simulink subsystem "ros_command"  (R2022a)
settings: Solver=VariableStepAuto  StartTime=0.0  StopTime=10.0  RelTol=1e-3
undefined symbols (not defined in the file): MPC, simulink
libraries: robotlib x42
settings Model: Creator=lamarre  LastModifiedBy=lamarre
settings DebuggingCC: UnconnectedInputMsg=warning  UnconnectedOutputMsg=warning  UnconnectedLineMsg=warning
settings RTWCC: DLArmComputeVersion=19.05

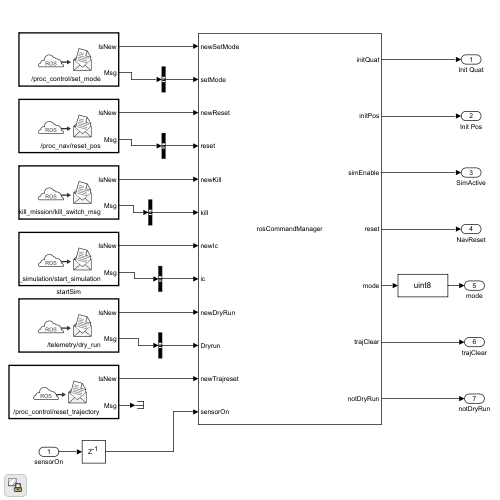
[thumbnail: Simulink's stored preview of the top-level diagram]
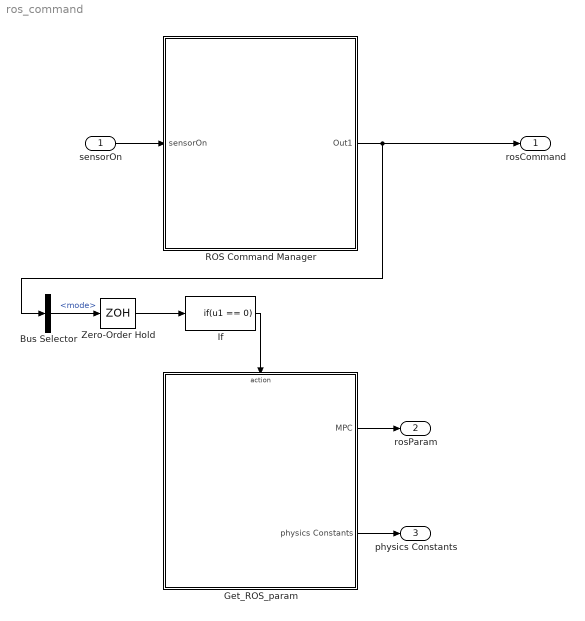
== system ros_command ==
  sensorOn : Inport
  Bus Selector : BusSelector  OutputSignals=mode
  "Get_ROS_param " : Subsystem
  If : If  IfExpression=u1 == 0  ShowElse=off
  ROS Command Manager : Subsystem  TreatAsAtomicUnit=on  SystemSampleTime=MPC.Ts
  Zero-Order Hold : ZeroOrderHold  SampleTime=simulink.ros.paramSampletime
  rosCommand : Outport
  rosParam : Outport  Port=2
  physics Constants : Outport  Port=3
  wires:
  sensorOn/1 -> ROS Command Manager/1(sensorOn)
  ROS Command Manager/1(Out1) -> rosCommand/1, Bus Selector/1
  If/1 -> "Get_ROS_param "/Action
  Bus Selector/1 -> Zero-Order Hold/1  "<mode>"
  "Get_ROS_param "/1(MPC) -> rosParam/1
  "Get_ROS_param "/2(physics Constants) -> physics Constants/1
  Zero-Order Hold/1 -> If/1

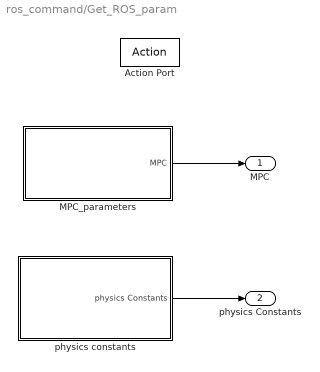
== system ros_command/Get_ROS_param  ==
  Action Port : ActionPort  InitializeStates=reset
  MPC_parameters : Subsystem
  physics constants : Subsystem
  MPC : Outport
  physics Constants : Outport  Port=2
  wires:
  physics constants/1(physics Constants) -> physics Constants/1
  MPC_parameters/1(MPC) -> MPC/1

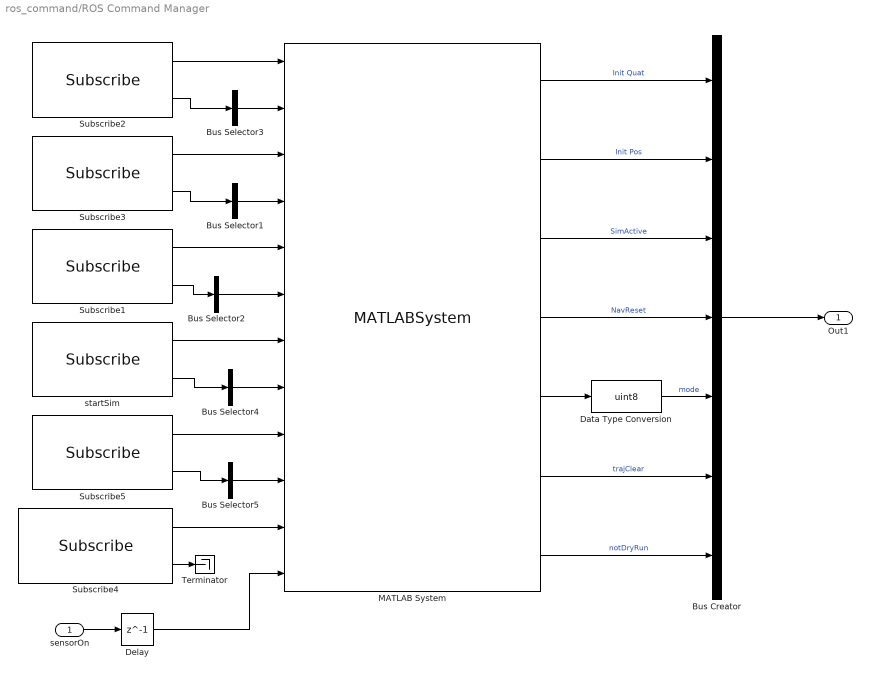
== system ros_command/ROS Command Manager ==
  sensorOn : Inport
  Bus Creator : BusCreator  Inputs=7
  Bus Selector{1..3,5} (4 alike) : BusSelector  OutputSignals=Data  OutputAsBus=on
  Bus Selector4 : BusSelector  OutputSignals=Position.X,Position.Y,Position.Z,Orientation.W,Orientation.X,Orientation.Y,Orientation.Z  OutputAsBus=on
  Data Type Conversion : DataTypeConversion  OutDataTypeStr=uint8  SaturateOnIntegerOverflow=off  RndMeth=Floor
  Delay : Delay  DelayLength=1  InitialCondition=0
  MATLAB System : MATLABSystem  System=rosCommandManager  initial_mode=mode.init  SimulateUsing=Code generation
      mask Type: rosCommandManager
      mask Display:
      | disp('rosCommandManager');
      | port_label('input',1,'newSetMode');
      | port_label('input',2,'setMode');
      | port_label('input',3,'newReset');
      | port_label('input',4,'reset');
      | port_label('input',5,'newKill');
      | port_label('input',6,'kill');
      | port_label('input',7,'newIc');
      | port_label('input',8,'ic');
      | port_label('input',9,'newDryRun');
      | port_label('input',10,'Dryrun');
      | port_label('input',11,'newTrajreset');
      | port_label('input',12,'sensorOn');
      | port_label('output',1,'initQuat');
      | port_label('output',2,'initPos');
      | port_label('output',3,'simEnable');
      | port_label('output',4,'reset');
      | port_label('output',5,'mode');
      | port_label('output',6,'trajClear');
      | port_label('output',7,'notDryRun');
  Subscribe1 : robotlib/Subscribe  topicSource=Specify your own  topic=/provider_kill_mission/kill_switch_msg  messageType=std_msgs/Bool  SampleTime=MPC.Ts  legacyBusStruct=off  messageQueueLength=1
  Subscribe2 : robotlib/Subscribe  topicSource=Specify your own  topic=/proc_control/set_mode  messageType=std_msgs/UInt8  SampleTime=MPC.Ts  legacyBusStruct=off  messageQueueLength=1
  Subscribe3 : robotlib/Subscribe  topicSource=Specify your own  topic=/proc_nav/reset_pos  messageType=std_msgs/Bool  SampleTime=MPC.Ts  legacyBusStruct=off  messageQueueLength=1
  Subscribe4 : robotlib/Subscribe  topicSource=Specify your own  topic=/proc_control/reset_trajectory  messageType=std_msgs/Bool  SampleTime=MPC.Ts  legacyBusStruct=off  messageQueueLength=1
  Subscribe5 : robotlib/Subscribe  topicSource=Specify your own  topic=/telemetry/dry_run  messageType=std_msgs/Bool  SampleTime=MPC.Ts  legacyBusStruct=off  messageQueueLength=1
  Terminator : Terminator
  startSim : robotlib/Subscribe  topicSource=Specify your own  topic=/proc_simulation/start_simulation  messageType=geometry_msgs/Pose  SampleTime=MPC.Ts  legacyBusStruct=off  messageQueueLength=1
  Out1 : Outport
  wires:
  Subscribe3/1 -> MATLAB System/3
  Bus Selector5/1 -> MATLAB System/10
  startSim/2 -> Bus Selector4/1
  Subscribe2/1 -> MATLAB System/1
  MATLAB System/4 -> Bus Creator/4  "NavReset"
  Subscribe4/1 -> MATLAB System/11
  Bus Selector2/1 -> MATLAB System/6
  Bus Creator/1 -> Out1/1
  Bus Selector4/1 -> MATLAB System/8
  Subscribe3/2 -> Bus Selector1/1
  MATLAB System/7 -> Bus Creator/7  "notDryRun"
  Data Type Conversion/1 -> Bus Creator/5  "mode"
  sensorOn/1 -> Delay/1
  Subscribe4/2 -> Terminator/1
  Bus Selector3/1 -> MATLAB System/2
  startSim/1 -> MATLAB System/7
  MATLAB System/3 -> Bus Creator/3  "SimActive"
  Subscribe5/2 -> Bus Selector5/1
  Subscribe1/1 -> MATLAB System/5
  Subscribe2/2 -> Bus Selector3/1
  Subscribe1/2 -> Bus Selector2/1
  Bus Selector1/1 -> MATLAB System/4
  Delay/1 -> MATLAB System/12
  Subscribe5/1 -> MATLAB System/9
  MATLAB System/6 -> Bus Creator/6  "trajClear"
  MATLAB System/2 -> Bus Creator/2  "Init Pos"
  MATLAB System/5 -> Data Type Conversion/1
  MATLAB System/1 -> Bus Creator/1  "Init Quat"

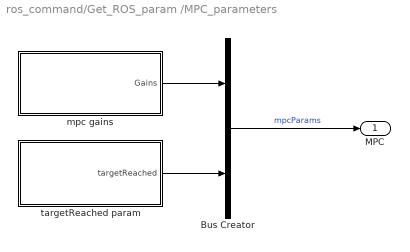
== system ros_command/Get_ROS_param /MPC_parameters ==
  Bus Creator : BusCreator  Inputs=2  OutDataTypeStr=Bus: mpcParams  NonVirtualBus=on
  mpc gains : Subsystem
  targetReached param : Subsystem
  MPC : Outport
  wires:
  Bus Creator/1 -> MPC/1  "mpcParams"
  mpc gains/1(Gains) -> Bus Creator/1
  targetReached param/1(targetReached) -> Bus Creator/2

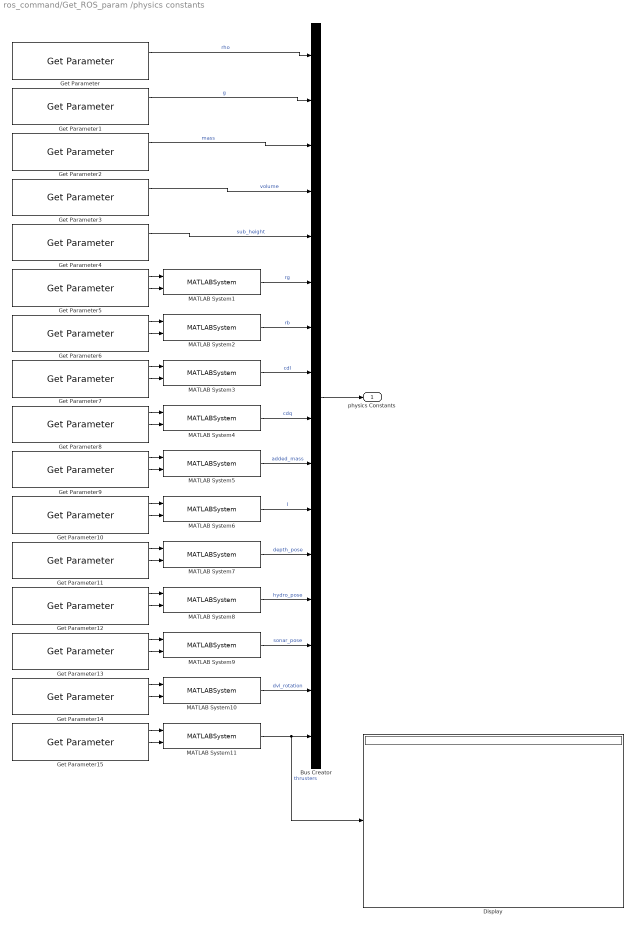
== system ros_command/Get_ROS_param /physics constants ==
  Bus Creator : BusCreator  Inputs=16  OutDataTypeStr=Bus: physicsConstants  NonVirtualBus=on
  Display : Display
  Get Parameter : robotlib/Get Parameter  ParameterSource=Specify your own  ParameterName=/proc_control/physics/rho  ParameterType=double  ParameterMaxArrayLength=16  ParameterInitialValue=physics.rho  SampleTime=-1  ShowErrorCodeOutput=on  ModelName=proc_control  BlockId=ParamGet_proc_control_185_535
      settings: SourceProductBaseCode=RR
  Get Parameter1 : robotlib/Get Parameter  ParameterSource=Specify your own  ParameterName=/proc_control/physics/g  ParameterType=double  ParameterMaxArrayLength=16  ParameterInitialValue=physics.g  SampleTime=-1  ShowErrorCodeOutput=on  ModelName=proc_control  BlockId=ParamGet_proc_control_185_540
      settings: SourceProductBaseCode=RR
  Get Parameter10 : robotlib/Get Parameter  ParameterSource=Specify your own  ParameterName=/proc_control/physics/I  ParameterType=uint8[] (string)  ParameterMaxArrayLength=128  ParameterInitialValue=int8('0,0,0,0,0,0,0,0,0')  SampleTime=-1  ShowErrorCodeOutput=on  ModelName=proc_control  BlockId=ParamGet_proc_control_185_554
      settings: SourceProductBaseCode=RR
  Get Parameter11 : robotlib/Get Parameter  ParameterSource=Specify your own  ParameterName=/proc_control/physics/depth_pose  ParameterType=uint8[] (string)  ParameterMaxArrayLength=64  ParameterInitialValue=int8('0,0,0')  SampleTime=-1  ShowErrorCodeOutput=on  ModelName=proc_control  BlockId=ParamGet_proc_control_185_556
      settings: SourceProductBaseCode=RR
  Get Parameter12 : robotlib/Get Parameter  ParameterSource=Specify your own  ParameterName=/proc_control/physics/hydro_pose  ParameterType=uint8[] (string)  ParameterMaxArrayLength=64  ParameterInitialValue=int8('0,0,0')  SampleTime=-1  ShowErrorCodeOutput=on  ModelName=proc_control  BlockId=ParamGet_proc_control_185_558
      settings: SourceProductBaseCode=RR
  Get Parameter13 : robotlib/Get Parameter  ParameterSource=Specify your own  ParameterName=/proc_control/physics/sonar_pose  ParameterType=uint8[] (string)  ParameterMaxArrayLength=64  ParameterInitialValue=int8('0,0,0')  SampleTime=-1  ShowErrorCodeOutput=on  ModelName=proc_control  BlockId=ParamGet_proc_control_185_560
      settings: SourceProductBaseCode=RR
  Get Parameter14 : robotlib/Get Parameter  ParameterSource=Specify your own  ParameterName=/proc_control/physics/dvl_rotation  ParameterType=uint8[] (string)  ParameterMaxArrayLength=64  ParameterInitialValue=int8('0,0,0')  SampleTime=-1  ShowErrorCodeOutput=on  ModelName=proc_control  BlockId=ParamGet_proc_control_185_562
      settings: SourceProductBaseCode=RR
  Get Parameter15 : robotlib/Get Parameter  ParameterSource=Specify your own  ParameterName=/proc_control/physics/thrusters  ParameterType=uint8[] (string)  ParameterMaxArrayLength=400  ParameterInitialValue=int8('0,0,0')  SampleTime=-1  ShowErrorCodeOutput=on  ModelName=proc_control  BlockId=ParamGet_proc_control_185_568
      settings: SourceProductBaseCode=RR
  Get Parameter2 : robotlib/Get Parameter  ParameterSource=Specify your own  ParameterName=/proc_control/physics/mass  ParameterType=double  ParameterMaxArrayLength=16  ParameterInitialValue=physics.mass  SampleTime=-1  ShowErrorCodeOutput=on  ModelName=proc_control  BlockId=ParamGet_proc_control_185_541
      settings: SourceProductBaseCode=RR
  Get Parameter3 : robotlib/Get Parameter  ParameterSource=Specify your own  ParameterName=/proc_control/physics/volume  ParameterType=double  ParameterMaxArrayLength=16  ParameterInitialValue=physics.volume  SampleTime=-1  ShowErrorCodeOutput=on  ModelName=proc_control  BlockId=ParamGet_proc_control_185_542
      settings: SourceProductBaseCode=RR
  Get Parameter4 : robotlib/Get Parameter  ParameterSource=Specify your own  ParameterName=/proc_control/physics/sub_height  ParameterType=double  ParameterMaxArrayLength=16  ParameterInitialValue=physics.height  SampleTime=-1  ShowErrorCodeOutput=on  ModelName=proc_control  BlockId=ParamGet_proc_control_185_543
      settings: SourceProductBaseCode=RR
  Get Parameter5 : robotlib/Get Parameter  ParameterSource=Specify your own  ParameterName=/proc_control/physics/rg  ParameterType=uint8[] (string)  ParameterMaxArrayLength=64  ParameterInitialValue=int8('0,0,0')  SampleTime=-1  ShowErrorCodeOutput=on  ModelName=proc_control  BlockId=ParamGet_proc_control_185_544
      settings: SourceProductBaseCode=RR
  Get Parameter6 : robotlib/Get Parameter  ParameterSource=Specify your own  ParameterName=/proc_control/physics/rb  ParameterType=uint8[] (string)  ParameterMaxArrayLength=64  ParameterInitialValue=int8('0,0,0')  SampleTime=-1  ShowErrorCodeOutput=on  ModelName=proc_control  BlockId=ParamGet_proc_control_185_546
      settings: SourceProductBaseCode=RR
  Get Parameter7 : robotlib/Get Parameter  ParameterSource=Specify your own  ParameterName=/proc_control/physics/cdl  ParameterType=uint8[] (string)  ParameterMaxArrayLength=64  ParameterInitialValue=int8('0,0,0,0,0,0')  SampleTime=-1  ShowErrorCodeOutput=on  ModelName=proc_control  BlockId=ParamGet_proc_control_185_548
      settings: SourceProductBaseCode=RR
  Get Parameter8 : robotlib/Get Parameter  ParameterSource=Specify your own  ParameterName=/proc_control/physics/cdq  ParameterType=uint8[] (string)  ParameterMaxArrayLength=64  ParameterInitialValue=int8('0,0,0,0,0,0')  SampleTime=-1  ShowErrorCodeOutput=on  ModelName=proc_control  BlockId=ParamGet_proc_control_185_549
      settings: SourceProductBaseCode=RR
  Get Parameter9 : robotlib/Get Parameter  ParameterSource=Specify your own  ParameterName=/proc_control/physics/added_mass  ParameterType=uint8[] (string)  ParameterMaxArrayLength=64  ParameterInitialValue=int8('0,0,0,0,0,0')  SampleTime=-1  ShowErrorCodeOutput=on  ModelName=proc_control  BlockId=ParamGet_proc_control_185_552
      settings: SourceProductBaseCode=RR
  MATLAB System1 : MATLABSystem  System=String2DoubleArray  arraySize=[1, 3]  constantName='Center of mass'  SimulateUsing=Code generation
      mask Type: String2DoubleArray
      mask Display:
      | disp('String2DoubleArray');
      | port_label('input',1,'string');
      | port_label('input',2,'length');
      | port_label('output',1,'array');
  MATLAB System10 : MATLABSystem  System=String2DoubleArray  arraySize=[1, 3]  constantName='DVL Rotation'  SimulateUsing=Code generation
      mask Type: String2DoubleArray
      mask Display:
      | disp('String2DoubleArray');
      | port_label('input',1,'string');
      | port_label('input',2,'length');
      | port_label('output',1,'array');
  MATLAB System11 : MATLABSystem  System=String2DoubleArray  arraySize=[MPC.nu 6]  constantName='Thrusters Config'  SimulateUsing=Code generation
      mask Type: String2DoubleArray
      mask Display:
      | disp('String2DoubleArray');
      | port_label('input',1,'string');
      | port_label('input',2,'length');
      | port_label('output',1,'array');
  MATLAB System2 : MATLABSystem  System=String2DoubleArray  arraySize=[1, 3]  constantName='Center of buoyancy'  SimulateUsing=Code generation
      mask Type: String2DoubleArray
      mask Display:
      | disp('String2DoubleArray');
      | port_label('input',1,'string');
      | port_label('input',2,'length');
      | port_label('output',1,'array');
  MATLAB System3 : MATLABSystem  System=String2DoubleArray  arraySize=[1,6]  constantName='Linear drag constants'  SimulateUsing=Code generation
      mask Type: String2DoubleArray
      mask Display:
      | disp('String2DoubleArray');
      | port_label('input',1,'string');
      | port_label('input',2,'length');
      | port_label('output',1,'array');
  MATLAB System4 : MATLABSystem  System=String2DoubleArray  arraySize=[1, 6]  constantName='Quadratic drag constants'  SimulateUsing=Code generation
      mask Type: String2DoubleArray
      mask Display:
      | disp('String2DoubleArray');
      | port_label('input',1,'string');
      | port_label('input',2,'length');
      | port_label('output',1,'array');
  MATLAB System5 : MATLABSystem  System=String2DoubleArray  arraySize=[1, 6]  constantName='Added Mass'  SimulateUsing=Code generation
      mask Type: String2DoubleArray
      mask Display:
      | disp('String2DoubleArray');
      | port_label('input',1,'string');
      | port_label('input',2,'length');
      | port_label('output',1,'array');
  MATLAB System6 : MATLABSystem  System=String2DoubleArray  arraySize=[1,9]  constantName='Inertia Tensor'  SimulateUsing=Code generation
      mask Type: String2DoubleArray
      mask Display:
      | disp('String2DoubleArray');
      | port_label('input',1,'string');
      | port_label('input',2,'length');
      | port_label('output',1,'array');
  MATLAB System7 : MATLABSystem  System=String2DoubleArray  arraySize=[1, 3]  constantName='Depth Pose'  SimulateUsing=Code generation
      mask Type: String2DoubleArray
      mask Display:
      | disp('String2DoubleArray');
      | port_label('input',1,'string');
      | port_label('input',2,'length');
      | port_label('output',1,'array');
  MATLAB System8 : MATLABSystem  System=String2DoubleArray  arraySize=[1, 3]  constantName='Hydro Pose'  SimulateUsing=Code generation
      mask Type: String2DoubleArray
      mask Display:
      | disp('String2DoubleArray');
      | port_label('input',1,'string');
      | port_label('input',2,'length');
      | port_label('output',1,'array');
  MATLAB System9 : MATLABSystem  System=String2DoubleArray  arraySize=[1, 3]  constantName='Sonar Pose'  SimulateUsing=Code generation
      mask Type: String2DoubleArray
      mask Display:
      | disp('String2DoubleArray');
      | port_label('input',1,'string');
      | port_label('input',2,'length');
      | port_label('output',1,'array');
  physics Constants : Outport
  wires:
  MATLAB System11/1 -> Bus Creator/16, Display/1  "thrusters"
  Get Parameter15/2 -> MATLAB System11/2
  Get Parameter15/1 -> MATLAB System11/1
  MATLAB System10/1 -> Bus Creator/15  "dvl_rotation"
  Get Parameter14/1 -> MATLAB System10/1
  Get Parameter14/2 -> MATLAB System10/2
  MATLAB System9/1 -> Bus Creator/14  "sonar_pose"
  Get Parameter13/1 -> MATLAB System9/1
  Get Parameter13/2 -> MATLAB System9/2
  MATLAB System8/1 -> Bus Creator/13  "hydro_pose"
  Get Parameter12/1 -> MATLAB System8/1
  Get Parameter12/2 -> MATLAB System8/2
  MATLAB System7/1 -> Bus Creator/12  "depth_pose"
  Get Parameter11/2 -> MATLAB System7/2
  Get Parameter11/1 -> MATLAB System7/1
  MATLAB System6/1 -> Bus Creator/11  "I"
  Get Parameter10/1 -> MATLAB System6/1
  Get Parameter10/2 -> MATLAB System6/2
  MATLAB System5/1 -> Bus Creator/10  "added_mass"
  Get Parameter9/1 -> MATLAB System5/1
  Get Parameter9/2 -> MATLAB System5/2
  MATLAB System4/1 -> Bus Creator/9  "cdq"
  MATLAB System3/1 -> Bus Creator/8  "cdl"
  Get Parameter8/2 -> MATLAB System4/2
  Get Parameter7/2 -> MATLAB System3/2
  Get Parameter7/1 -> MATLAB System3/1
  Get Parameter8/1 -> MATLAB System4/1
  MATLAB System2/1 -> Bus Creator/7  "rb"
  Get Parameter6/2 -> MATLAB System2/2
  Get Parameter6/1 -> MATLAB System2/1
  MATLAB System1/1 -> Bus Creator/6  "rg"
  Get Parameter5/2 -> MATLAB System1/2
  Get Parameter5/1 -> MATLAB System1/1
  Get Parameter4/1 -> Bus Creator/5  "sub_height"
  Get Parameter3/1 -> Bus Creator/4  "volume"
  Get Parameter2/1 -> Bus Creator/3  "mass"
  Get Parameter1/1 -> Bus Creator/2  "g"
  Bus Creator/1 -> physics Constants/1
  Get Parameter/1 -> Bus Creator/1  "rho"

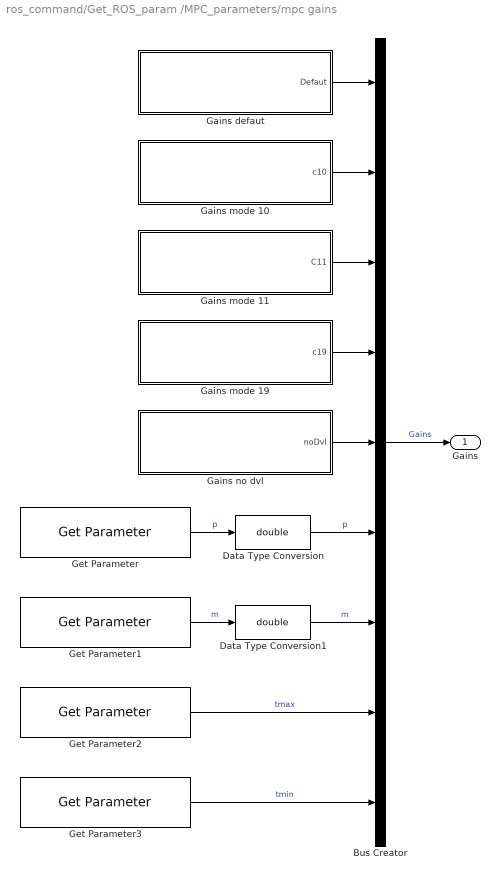
== system ros_command/Get_ROS_param /MPC_parameters/mpc gains ==
  Bus Creator : BusCreator  Inputs=9
  Data Type Conversion : DataTypeConversion  OutDataTypeStr=double  SaturateOnIntegerOverflow=off  RndMeth=Floor
  Data Type Conversion1 : DataTypeConversion  OutDataTypeStr=double  SaturateOnIntegerOverflow=off  RndMeth=Floor
  Gains defaut : Subsystem
  Gains mode 10 : Subsystem
  Gains mode 11 : Subsystem
  Gains mode 19 : Subsystem
  Gains no dvl : Subsystem
  Get Parameter : robotlib/Get Parameter  ParameterSource=Specify your own  ParameterName=/proc_control/mpc/p  ParameterType=int32  ParameterMaxArrayLength=16  ParameterInitialValue=MPC.p  SampleTime=-1  ShowErrorCodeOutput=off  ModelName=proc_control  BlockId=ParamGet_proc_control_185_529
      settings: SourceProductBaseCode=RR
  Get Parameter1 : robotlib/Get Parameter  ParameterSource=Specify your own  ParameterName=/proc_control/mpc/m  ParameterType=int32  ParameterMaxArrayLength=16  ParameterInitialValue=MPC.m  SampleTime=-1  ShowErrorCodeOutput=off  ModelName=proc_control  BlockId=ParamGet_proc_control_185_530
      settings: SourceProductBaseCode=RR
  Get Parameter2 : robotlib/Get Parameter  ParameterSource=Specify your own  ParameterName=/proc_control/mpc/tmax  ParameterType=double  ParameterMaxArrayLength=16  ParameterInitialValue=MPC.tmax  SampleTime=-1  ShowErrorCodeOutput=off  ModelName=proc_control  BlockId=ParamGet_proc_control_185_533
      settings: SourceProductBaseCode=RR
  Get Parameter3 : robotlib/Get Parameter  ParameterSource=Specify your own  ParameterName=/proc_control/mpc/tmin  ParameterType=double  ParameterMaxArrayLength=16  ParameterInitialValue=MPC.tmin  SampleTime=-1  ShowErrorCodeOutput=off  ModelName=proc_control  BlockId=ParamGet_proc_control_185_534
      settings: SourceProductBaseCode=RR
  Gains : Outport
  wires:
  Get Parameter3/1 -> Bus Creator/9  "tmin"
  Get Parameter2/1 -> Bus Creator/8  "tmax"
  Get Parameter1/1 -> Data Type Conversion1/1  "m"
  Get Parameter/1 -> Data Type Conversion/1  "p"
  Data Type Conversion1/1 -> Bus Creator/7  "m"
  Data Type Conversion/1 -> Bus Creator/6  "p"
  Gains no dvl/1(noDvl) -> Bus Creator/5
  Gains defaut/1(Defaut) -> Bus Creator/1
  Gains mode 10/1(c10) -> Bus Creator/2
  Bus Creator/1 -> Gains/1  "Gains"
  Gains mode 19/1(c19) -> Bus Creator/4
  Gains mode 11/1(C11) -> Bus Creator/3

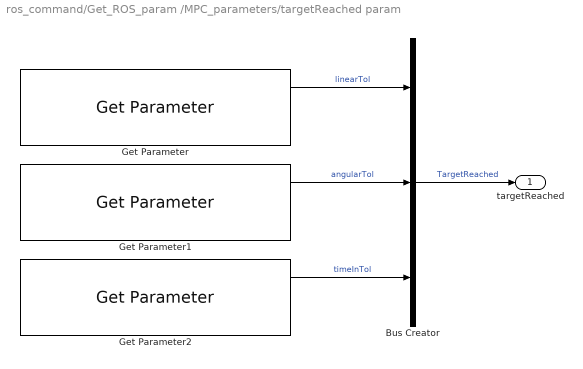
== system ros_command/Get_ROS_param /MPC_parameters/targetReached param ==
  Bus Creator : BusCreator  Inputs=3
  Get Parameter : robotlib/Get Parameter  ParameterSource=Specify your own  ParameterName=/proc_control/target_reached/linear_tolerance  ParameterType=double  ParameterMaxArrayLength=64  ParameterInitialValue=MPC.targetReached.linearTol  SampleTime=-1  ShowErrorCodeOutput=on  ModelName=proc_control  BlockId=ParamGet_proc_control_185_503
      settings: SourceProductBaseCode=RR
  Get Parameter1 : robotlib/Get Parameter  ParameterSource=Specify your own  ParameterName=/proc_control/target_reached/angular_tolerance  ParameterType=double  ParameterMaxArrayLength=64  ParameterInitialValue=MPC.targetReached.angularTol  SampleTime=-1  ShowErrorCodeOutput=on  ModelName=proc_control  BlockId=ParamGet_proc_control_185_504
      settings: SourceProductBaseCode=RR
  Get Parameter2 : robotlib/Get Parameter  ParameterSource=Specify your own  ParameterName=/proc_control/target_reached/time_in_tolerance  ParameterType=double  ParameterMaxArrayLength=64  ParameterInitialValue=MPC.targetReached.timeInTol  SampleTime=-1  ShowErrorCodeOutput=on  ModelName=proc_control  BlockId=ParamGet_proc_control_185_505
      settings: SourceProductBaseCode=RR
  targetReached : Outport
  wires:
  Bus Creator/1 -> targetReached/1  "TargetReached"
  Get Parameter1/1 -> Bus Creator/2  "angularTol"
  Get Parameter/1 -> Bus Creator/1  "linearTol"
  Get Parameter2/1 -> Bus Creator/3  "timeInTol"

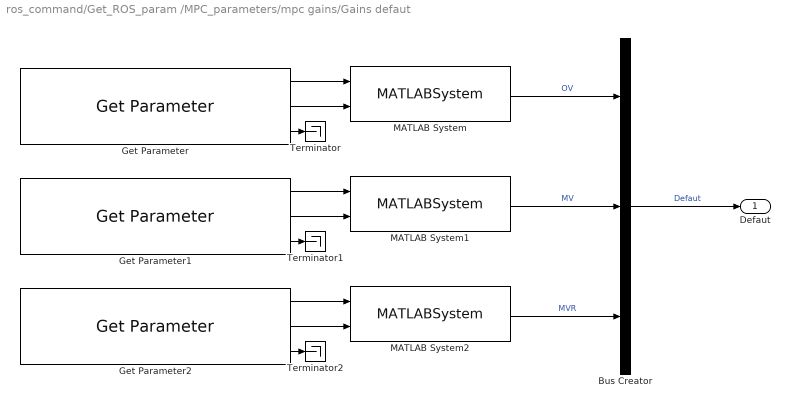
== system ros_command/Get_ROS_param /MPC_parameters/mpc gains/Gains defaut ==
  Bus Creator : BusCreator  Inputs=3
  Get Parameter : robotlib/Get Parameter  ParameterSource=Specify your own  ParameterName=/proc_control/mpc/gains/default/ov  ParameterType=uint8[] (string)  ParameterMaxArrayLength=64  ParameterInitialValue=uint8('30,30,30,45,45,45,45,0,0,0,0,0,0')  SampleTime=-1  ShowErrorCodeOutput=on  ModelName=proc_control  BlockId=ParamGet_proc_control_185_465
      settings: SourceProductBaseCode=RR
  Get Parameter1 : robotlib/Get Parameter  ParameterSource=Specify your own  ParameterName=/proc_control/mpc/gains/default/mv  ParameterType=uint8[] (string)  ParameterMaxArrayLength=64  ParameterInitialValue=uint8('30,30,30,45,45,45,45,0,0,0,0,0,0')  SampleTime=-1  ShowErrorCodeOutput=on  ModelName=proc_control  BlockId=ParamGet_proc_control_185_466
      settings: SourceProductBaseCode=RR
  Get Parameter2 : robotlib/Get Parameter  ParameterSource=Specify your own  ParameterName=/proc_control/mpc/gains/default/mvr  ParameterType=uint8[] (string)  ParameterMaxArrayLength=64  ParameterInitialValue=uint8('30,30,30,45,45,45,45,0,0,0,0,0,0')  SampleTime=-1  ShowErrorCodeOutput=on  ModelName=proc_control  BlockId=ParamGet_proc_control_185_467
      settings: SourceProductBaseCode=RR
  MATLAB System : MATLABSystem  System=String2DoubleArray  arraySize=[1 MPC.nx]  constantName='Default OV'  SimulateUsing=Code generation
      mask Type: String2DoubleArray
      mask Display:
      | disp('String2DoubleArray');
      | port_label('input',1,'string');
      | port_label('input',2,'length');
      | port_label('output',1,'array');
  MATLAB System1 : MATLABSystem  System=String2DoubleArray  arraySize=[1 MPC.nu]  constantName='Default MV'  SimulateUsing=Code generation
      mask Type: String2DoubleArray
      mask Display:
      | disp('String2DoubleArray');
      | port_label('input',1,'string');
      | port_label('input',2,'length');
      | port_label('output',1,'array');
  MATLAB System2 : MATLABSystem  System=String2DoubleArray  arraySize=[1 MPC.nu]  constantName='Default MVR'  SimulateUsing=Code generation
      mask Type: String2DoubleArray
      mask Display:
      | disp('String2DoubleArray');
      | port_label('input',1,'string');
      | port_label('input',2,'length');
      | port_label('output',1,'array');
  Terminator : Terminator
  Terminator1 : Terminator
  Terminator2 : Terminator
  Defaut : Outport
  wires:
  Get Parameter2/3 -> Terminator2/1
  Get Parameter1/3 -> Terminator1/1
  MATLAB System2/1 -> Bus Creator/3  "MVR"
  MATLAB System/1 -> Bus Creator/1  "OV"
  Get Parameter/1 -> MATLAB System/1
  Bus Creator/1 -> Defaut/1  "Defaut"
  Get Parameter1/1 -> MATLAB System1/1
  Get Parameter/3 -> Terminator/1
  Get Parameter2/2 -> MATLAB System2/2
  MATLAB System1/1 -> Bus Creator/2  "MV"
  Get Parameter1/2 -> MATLAB System1/2
  Get Parameter/2 -> MATLAB System/2
  Get Parameter2/1 -> MATLAB System2/1

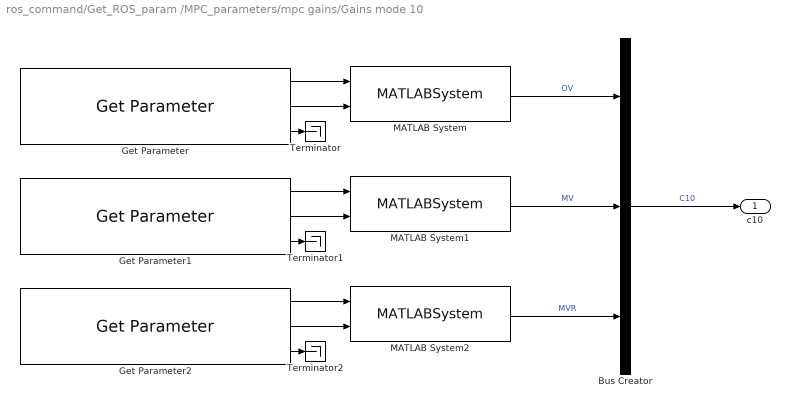
== system ros_command/Get_ROS_param /MPC_parameters/mpc gains/Gains mode 10 ==
  Bus Creator : BusCreator  Inputs=3
  Get Parameter : robotlib/Get Parameter  ParameterSource=Specify your own  ParameterName=/proc_control/mpc/gains/c10/ov  ParameterType=uint8[] (string)  ParameterMaxArrayLength=64  ParameterInitialValue=uint8('30,30,30,45,45,45,45,0,0,0,0,0,0')  SampleTime=-1  ShowErrorCodeOutput=on  ModelName=proc_control  BlockId=ParamGet_proc_control_185_440
      settings: SourceProductBaseCode=RR
  Get Parameter1 : robotlib/Get Parameter  ParameterSource=Specify your own  ParameterName=/proc_control/mpc/gains/c10/mv  ParameterType=uint8[] (string)  ParameterMaxArrayLength=64  ParameterInitialValue=uint8('30,30,30,45,45,45,45,0,0,0,0,0,0')  SampleTime=-1  ShowErrorCodeOutput=on  ModelName=proc_control  BlockId=ParamGet_proc_control_185_441
      settings: SourceProductBaseCode=RR
  Get Parameter2 : robotlib/Get Parameter  ParameterSource=Specify your own  ParameterName=/proc_control/mpc/gains/c10/mvr  ParameterType=uint8[] (string)  ParameterMaxArrayLength=64  ParameterInitialValue=uint8('30,30,30,45,45,45,45,0,0,0,0,0,0')  SampleTime=-1  ShowErrorCodeOutput=on  ModelName=proc_control  BlockId=ParamGet_proc_control_185_442
      settings: SourceProductBaseCode=RR
  MATLAB System : MATLABSystem  System=String2DoubleArray  arraySize=[1 MPC.nx]  constantName='mode 10 OV'  SimulateUsing=Code generation
      mask Type: String2DoubleArray
      mask Display:
      | disp('String2DoubleArray');
      | port_label('input',1,'string');
      | port_label('input',2,'length');
      | port_label('output',1,'array');
  MATLAB System1 : MATLABSystem  System=String2DoubleArray  arraySize=[1 MPC.nu]  constantName='mode 10 MV'  SimulateUsing=Code generation
      mask Type: String2DoubleArray
      mask Display:
      | disp('String2DoubleArray');
      | port_label('input',1,'string');
      | port_label('input',2,'length');
      | port_label('output',1,'array');
  MATLAB System2 : MATLABSystem  System=String2DoubleArray  arraySize=[1 MPC.nu]  constantName='mode 10 MVR'  SimulateUsing=Code generation
      mask Type: String2DoubleArray
      mask Display:
      | disp('String2DoubleArray');
      | port_label('input',1,'string');
      | port_label('input',2,'length');
      | port_label('output',1,'array');
  Terminator : Terminator
  Terminator1 : Terminator
  Terminator2 : Terminator
  c10 : Outport
  wires:
  Get Parameter2/3 -> Terminator2/1
  Get Parameter1/3 -> Terminator1/1
  MATLAB System2/1 -> Bus Creator/3  "MVR"
  MATLAB System/1 -> Bus Creator/1  "OV"
  Get Parameter/1 -> MATLAB System/1
  Bus Creator/1 -> c10/1  "C10"
  Get Parameter1/1 -> MATLAB System1/1
  Get Parameter/3 -> Terminator/1
  Get Parameter2/2 -> MATLAB System2/2
  MATLAB System1/1 -> Bus Creator/2  "MV"
  Get Parameter1/2 -> MATLAB System1/2
  Get Parameter/2 -> MATLAB System/2
  Get Parameter2/1 -> MATLAB System2/1

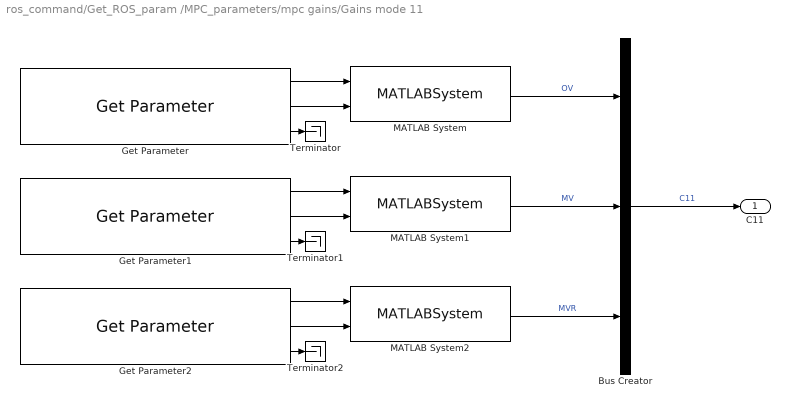
== system ros_command/Get_ROS_param /MPC_parameters/mpc gains/Gains mode 11 ==
  Bus Creator : BusCreator  Inputs=3
  Get Parameter : robotlib/Get Parameter  ParameterSource=Specify your own  ParameterName=/proc_control/mpc/gains/c11/ov  ParameterType=uint8[] (string)  ParameterMaxArrayLength=64  ParameterInitialValue=uint8('30,30,30,45,45,45,45,0,0,0,0,0,0')  SampleTime=-1  ShowErrorCodeOutput=on  ModelName=proc_control  BlockId=ParamGet_proc_control_185_453
      settings: SourceProductBaseCode=RR
  Get Parameter1 : robotlib/Get Parameter  ParameterSource=Specify your own  ParameterName=/proc_control/mpc/gains/c11/mv  ParameterType=uint8[] (string)  ParameterMaxArrayLength=64  ParameterInitialValue=uint8('30,30,30,45,45,45,45,0,0,0,0,0,0')  SampleTime=-1  ShowErrorCodeOutput=on  ModelName=proc_control  BlockId=ParamGet_proc_control_185_454
      settings: SourceProductBaseCode=RR
  Get Parameter2 : robotlib/Get Parameter  ParameterSource=Specify your own  ParameterName=/proc_control/mpc/gains/c11/mvr  ParameterType=uint8[] (string)  ParameterMaxArrayLength=64  ParameterInitialValue=uint8('30,30,30,45,45,45,45,0,0,0,0,0,0')  SampleTime=-1  ShowErrorCodeOutput=on  ModelName=proc_control  BlockId=ParamGet_proc_control_185_455
      settings: SourceProductBaseCode=RR
  MATLAB System : MATLABSystem  System=String2DoubleArray  arraySize=[1 MPC.nx]  constantName='mode 11 OV'  SimulateUsing=Code generation
      mask Type: String2DoubleArray
      mask Display:
      | disp('String2DoubleArray');
      | port_label('input',1,'string');
      | port_label('input',2,'length');
      | port_label('output',1,'array');
  MATLAB System1 : MATLABSystem  System=String2DoubleArray  arraySize=[1 MPC.nu]  constantName='mode 11 MV'  SimulateUsing=Code generation
      mask Type: String2DoubleArray
      mask Display:
      | disp('String2DoubleArray');
      | port_label('input',1,'string');
      | port_label('input',2,'length');
      | port_label('output',1,'array');
  MATLAB System2 : MATLABSystem  System=String2DoubleArray  arraySize=[1 MPC.nu]  constantName='mode 11 MVR'  SimulateUsing=Code generation
      mask Type: String2DoubleArray
      mask Display:
      | disp('String2DoubleArray');
      | port_label('input',1,'string');
      | port_label('input',2,'length');
      | port_label('output',1,'array');
  Terminator : Terminator
  Terminator1 : Terminator
  Terminator2 : Terminator
  C11 : Outport
  wires:
  Get Parameter2/3 -> Terminator2/1
  Get Parameter1/3 -> Terminator1/1
  MATLAB System2/1 -> Bus Creator/3  "MVR"
  MATLAB System/1 -> Bus Creator/1  "OV"
  Get Parameter/1 -> MATLAB System/1
  Bus Creator/1 -> C11/1  "C11"
  Get Parameter1/1 -> MATLAB System1/1
  Get Parameter/3 -> Terminator/1
  Get Parameter2/2 -> MATLAB System2/2
  MATLAB System1/1 -> Bus Creator/2  "MV"
  Get Parameter1/2 -> MATLAB System1/2
  Get Parameter/2 -> MATLAB System/2
  Get Parameter2/1 -> MATLAB System2/1

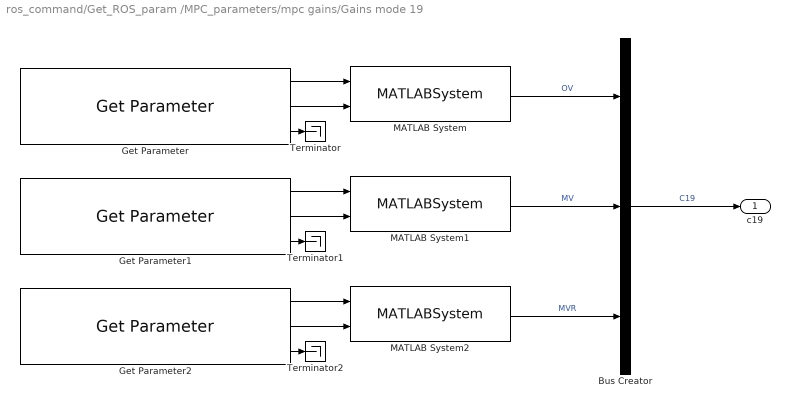
== system ros_command/Get_ROS_param /MPC_parameters/mpc gains/Gains mode 19 ==
  Bus Creator : BusCreator  Inputs=3
  Get Parameter : robotlib/Get Parameter  ParameterSource=Specify your own  ParameterName=/proc_control/mpc/gains/c19/ov  ParameterType=uint8[] (string)  ParameterMaxArrayLength=64  ParameterInitialValue=uint8('30,30,30,45,45,45,45,0,0,0,0,0,0')  SampleTime=-1  ShowErrorCodeOutput=on  ModelName=proc_control  BlockId=ParamGet_proc_control_185_477
      settings: SourceProductBaseCode=RR
  Get Parameter1 : robotlib/Get Parameter  ParameterSource=Specify your own  ParameterName=/proc_control/mpc/gains/c19/mv  ParameterType=uint8[] (string)  ParameterMaxArrayLength=64  ParameterInitialValue=uint8('30,30,30,45,45,45,45,0,0,0,0,0,0')  SampleTime=-1  ShowErrorCodeOutput=on  ModelName=proc_control  BlockId=ParamGet_proc_control_185_478
      settings: SourceProductBaseCode=RR
  Get Parameter2 : robotlib/Get Parameter  ParameterSource=Specify your own  ParameterName=/proc_control/mpc/gains/c19/mvr  ParameterType=uint8[] (string)  ParameterMaxArrayLength=64  ParameterInitialValue=uint8('30,30,30,45,45,45,45,0,0,0,0,0,0')  SampleTime=-1  ShowErrorCodeOutput=on  ModelName=proc_control  BlockId=ParamGet_proc_control_185_479
      settings: SourceProductBaseCode=RR
  MATLAB System : MATLABSystem  System=String2DoubleArray  arraySize=[1 MPC.nx]  constantName='mode 19 OV'  SimulateUsing=Code generation
      mask Type: String2DoubleArray
      mask Display:
      | disp('String2DoubleArray');
      | port_label('input',1,'string');
      | port_label('input',2,'length');
      | port_label('output',1,'array');
  MATLAB System1 : MATLABSystem  System=String2DoubleArray  arraySize=[1 MPC.nu]  constantName='mode 19 MV'  SimulateUsing=Code generation
      mask Type: String2DoubleArray
      mask Display:
      | disp('String2DoubleArray');
      | port_label('input',1,'string');
      | port_label('input',2,'length');
      | port_label('output',1,'array');
  MATLAB System2 : MATLABSystem  System=String2DoubleArray  arraySize=[1 MPC.nu]  constantName='mode 19 MVR'  SimulateUsing=Code generation
      mask Type: String2DoubleArray
      mask Display:
      | disp('String2DoubleArray');
      | port_label('input',1,'string');
      | port_label('input',2,'length');
      | port_label('output',1,'array');
  Terminator : Terminator
  Terminator1 : Terminator
  Terminator2 : Terminator
  c19 : Outport
  wires:
  Get Parameter2/3 -> Terminator2/1
  Get Parameter1/3 -> Terminator1/1
  MATLAB System2/1 -> Bus Creator/3  "MVR"
  MATLAB System/1 -> Bus Creator/1  "OV"
  Get Parameter/1 -> MATLAB System/1
  Bus Creator/1 -> c19/1  "C19"
  Get Parameter1/1 -> MATLAB System1/1
  Get Parameter/3 -> Terminator/1
  Get Parameter2/2 -> MATLAB System2/2
  MATLAB System1/1 -> Bus Creator/2  "MV"
  Get Parameter1/2 -> MATLAB System1/2
  Get Parameter/2 -> MATLAB System/2
  Get Parameter2/1 -> MATLAB System2/1

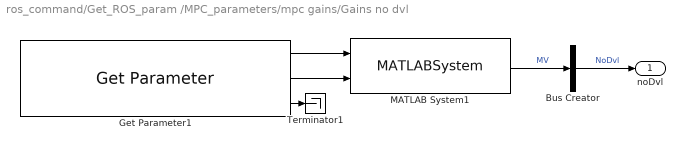
== system ros_command/Get_ROS_param /MPC_parameters/mpc gains/Gains no dvl ==
  Bus Creator : BusCreator  Inputs=1
  Get Parameter1 : robotlib/Get Parameter  ParameterSource=Specify your own  ParameterName=/proc_control/mpc/gains/noDvl/mv  ParameterType=uint8[] (string)  ParameterMaxArrayLength=64  ParameterInitialValue=uint8('30,30,30,45,45,45,45,0,0,0,0,0,0')  SampleTime=-1  ShowErrorCodeOutput=on  ModelName=proc_control  BlockId=ParamGet_proc_control_185_494
      settings: SourceProductBaseCode=RR
  MATLAB System1 : MATLABSystem  System=String2DoubleArray  arraySize=[1 MPC.nu]  constantName='no DVL MV'  SimulateUsing=Code generation
      mask Type: String2DoubleArray
      mask Display:
      | disp('String2DoubleArray');
      | port_label('input',1,'string');
      | port_label('input',2,'length');
      | port_label('output',1,'array');
  Terminator1 : Terminator
  noDvl : Outport
  wires:
  MATLAB System1/1 -> Bus Creator/1  "MV"
  Get Parameter1/3 -> Terminator1/1
  Bus Creator/1 -> noDvl/1  "NoDvl"
  Get Parameter1/1 -> MATLAB System1/1
  Get Parameter1/2 -> MATLAB System1/2
